simulink model "VCU_SW_1"  (R2023b)
settings: Solver=FixedStepDiscrete  StartTime=0.0  StopTime=inf  FixedStep=1e-2  RelTol=1e-3
PreLoadFcn:
  | RTWConfigurationCB('preloadfcn', bdroot);
InitFcn:
  | loadvar_ttc500
undefined symbols (not defined in the file): BrkPedalTypes, CabMovModeTypes, cFuseTempSensAcc_X, cFuseTempSensAcc_Y, cFuseTempSensVal_X, cFuseTempSensVal_Y, cTMSTempSensVal_X, cTMSTempSensVal_Y, cTransferCaseSpeedRatio, diag_state, DoorsPositionTypes, dP_filter_Y, DriverOccClassSystemTypes, ErrorValueTypes, fatal_error_callback, IO_ADC_NO_RANGE, LadderStatusTypes, pAnalogCabRotSensAcc, pAnalogCabRotSensMaxVolt, pAnalogCabRotSensMinVolt, pAnalogCabRotSensRange, pAnalogCabRotSensZeroVolt, pBrkActivePress, pCabTiltSensAcc, pCabTiltSensMaxCur, pCabTiltSensMinCur, pDistanceCorrection, pECANManual_BPNEnable, pECANManual_BPNEnabler_Flag, pFilterSensAccRes, pHDirMaxDiffFrq, pHDirSensHighLvl, pHDirSensLowLvl, pMainGearRatio, pMaxFilterSensRes, pMaxFirstPedalSensValue, pMaxFuseTempSensRes, pMaxPressLoss, pMaxPressSensCurrent, pMaxPressValue, pMaxPressValueHydMotAndPump, pMaxPressValueParkDrain, pMaxSecondPedalSensValue, pMaxTempSensVoltage, pMaxTempValue, pMaxTMSTempSensRes, pMinFilterSensRes, pMinFirstPedalSensValue, pMinFuseTempSensRes, pMinPressLoss, pMinPressSensCurrent, pMinPressValue, pMinSecondPedalSensValue, pMinTempSensVoltage, pMinTempValue, pMinTMSTempSensRes, pMotorRingTeethNum, pPedalSensAccuracyPct, pPedalSensAccuracyVolt, pPressLossTreshhold ... (+20)
libraries: TTlibrary x270, canmsglib x127, simulink x88
(part 10 of 19)

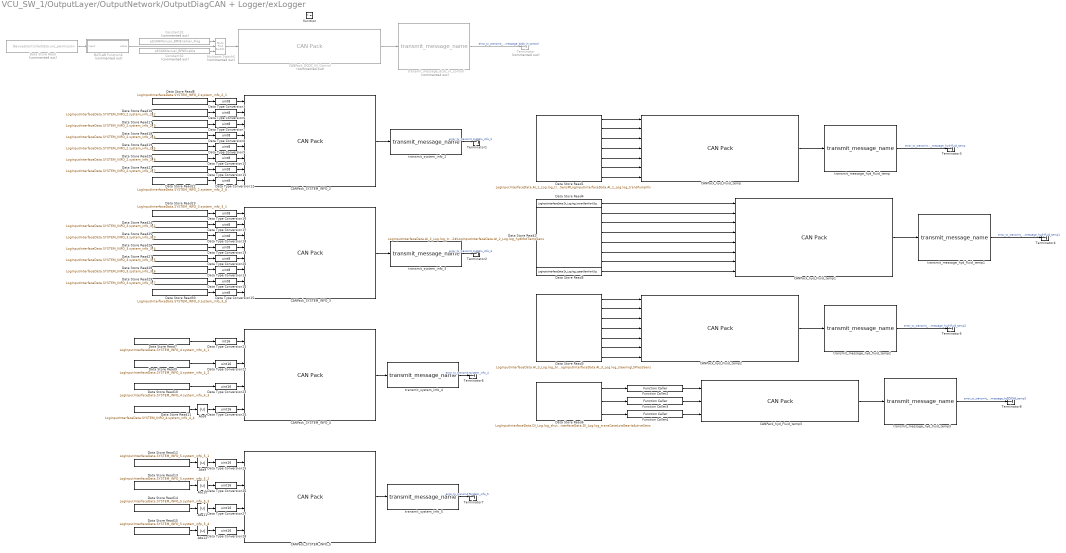
== system VCU_SW_1/OutputLayer/OutputNetwork/OutputDiagCAN + Logger/exLogger ==
  function : TriggerPort  TriggerType=function-call  VariantControl=Variant
  Abs{8..12} (5 alike) : Abs  SaturateOnIntegerOverflow=off
  CANPack_DCDC_IN_Control : canmsglib/CAN Pack  Commented=on  CANdbFile=C:\Users\shevchenko\Desktop\HerculesLittle\HerculesLittle\database\ElectricCAN.dbc  MsgList=(none)  MsgName=DCDC_IN_Control  MsgIDType=Extended (29-bit identifier)  MsgIdentifier=73  MsgLength=8  Remote=off  ApplyMinMax=off  BusOutput=on  SignalInfo={'BPN_Enable','0','1','LE','unsigned','Standard','0','1','0','0','1'}
      settings: DataFormat=CANdb specified signals
  CANPack_SYSTEM_INFO_2 : canmsglib/CAN Pack  MsgList=(none)  MsgName=SYSTEM_INFO_2  MsgIDType=Extended (29-bit identifier)  MsgIdentifier=419387898  MsgLength=8  Remote=off  ApplyMinMax=off  BusOutput=on  SignalInfo={ 'system_info_2_1', '0', '8', 'LE', 'unsigned', 'Standard', '0', '1', '0', '0', '255'; 'system_info_2_2', '8', '8', 'LE', 'unsigned', 'Standard', '0', '1', '0', '0', '255'; 'system_info_2_3', '16', '8', 'LE', 'unsigned', 'Standard', '0', '1', '0', '0', '255'; 'system_info_2_4', '24', '8', 'LE', 'unsigned', 'Standard', '0', '1', '0', '0', '255'; 'system_info_2_5', '32', '8', 'LE', 'unsigned', 'Standard', '0', '1', '0', '0', '255'; 'system_info_2_6', '40', '8', 'LE', 'unsigned', 'Standard', '0', '1', '0', '0', '255'; 'system_info_2_7', '48', '8', 'LE', 'unsigned', 'Standard', '0', '1', '0', '0', '255'; 'system_info_2_8', '56', '8', 'LE', 'unsigned', 'Standard', '0', '1', '0', '0', '255' }
      settings: DataFormat=manually specified signals
  CANPack_SYSTEM_INFO_3 : canmsglib/CAN Pack  MsgList=(none)  MsgName=SYSTEM_INFO_3  MsgIDType=Extended (29-bit identifier)  MsgIdentifier=419389690  MsgLength=8  Remote=off  ApplyMinMax=off  BusOutput=on  SignalInfo={ 'system_info_3_1', '0', '8', 'LE', 'unsigned', 'Standard', '0', '1', '0', '0', '255'; 'system_info_3_2', '8', '8', 'LE', 'unsigned', 'Standard', '0', '1', '0', '0', '255'; 'system_info_3_3', '16', '8', 'LE', 'unsigned', 'Standard', '0', '1', '0', '0', '255'; 'system_info_3_4', '24', '8', 'LE', 'unsigned', 'Standard', '0', '1', '0', '0', '255'; 'system_info_3_5', '32', '8', 'LE', 'unsigned', 'Standard', '0', '1', '0', '0', '255'; 'system_info_3_6', '40', '8', 'LE', 'unsigned', 'Standard', '0', '1', '0', '0', '255'; 'system_info_3_7', '48', '8', 'LE', 'unsigned', 'Standard', '0', '1', '0', '0', '255'; 'system_info_3_8', '56', '8', 'LE', 'unsigned', 'Standard', '0', '1', '0', '0', '255' }
      settings: DataFormat=manually specified signals
  CANPack_SYSTEM_INFO_4 : canmsglib/CAN Pack  MsgList=(none)  MsgName=SYSTEM_INFO_4  MsgIDType=Extended (29-bit identifier)  MsgIdentifier=419389946  MsgLength=8  Remote=off  ApplyMinMax=off  BusOutput=on  SignalInfo={ 'system_info_4_1', '0', '16', 'LE', 'unsigned', 'Standard', '0', '1', '-32768', '0', '32767'; 'system_info_4_2', '16', '16', 'LE', 'unsigned', 'Standard', '0', '1', '0', '0', '65535'; 'system_info_4_3', '32', '16', 'LE', 'unsigned', 'Standard', '0', '1', '0', '0', '65535'; 'system_info_4_4', '48', '16', 'LE', 'unsigned', 'Standard', '0', '1', '0', '0', '65535' }
      settings: DataFormat=manually specified signals
  CANPack_SYSTEM_INFO_5 : canmsglib/CAN Pack  MsgList=(none)  MsgName=SYSTEM_INFO_5  MsgIDType=Extended (29-bit identifier)  MsgIdentifier=419390202  MsgLength=8  Remote=off  ApplyMinMax=off  BusOutput=on  SignalInfo={ 'system_info_5_1', '0', '16', 'LE', 'unsigned', 'Standard', '0', '1', '0', '0', '65535'; 'system_info_5_2', '16', '16', 'LE', 'unsigned', 'Standard', '0', '1', '0', '0', '65535'; 'system_info_5_3', '32', '16', 'LE', 'unsigned', 'Standard', '0', '1', '0', '0', '65535'; 'system_info_5_4', '48', '16', 'LE', 'unsigned', 'Standard', '0', '1', '0', '0', '65535' }
      settings: DataFormat=manually specified signals
  CANPack_hyd_Fluid_temp : canmsglib/CAN Pack  MsgList=(none)  MsgName=Log_AI_1  MsgIDType=Extended (29-bit identifier)  MsgIdentifier=402657831  MsgLength=8  Remote=off  ApplyMinMax=off  BusOutput=on  SignalInfo={ 'TrHydPumpDirectSens', '24', '8', 'LE', 'unsigned', 'Standard', '0', '1', '0', '0', '255'; 'TrHydPumpFilterClogSens', '8', '8', 'LE', 'unsigned', 'Standard', '0', '2', '0', '0', '510'; 'TrHydPumpSpeedSens1', '32', '8', 'LE', 'unsigned', 'Standard', '0', '50', '0', '0', '12750'; 'TrHydPumpSpeedSens2', '16', '8', 'LE', 'unsigned', 'Standard', '0', '50', '0', '0', '12750'; 'TrHydPumpTempSens', '40', '8', 'LE', 'unsigned', 'Standard', '0', '10', '0', '0', '2550'; 'TrHydPumpWasherTiltSens', '0', '8', 'LE', 'unsigned', 'Standard', '0', '20', '0', '0', '5100'; 'TransmissionMotorHydDistr', '48', '8', 'LE', 'unsigned', 'Standard', '0', '4', '0', '0', '1020' }
      settings: DataFormat=manually specified signals
  CANPack_hyd_Fluid_temp1 : canmsglib/CAN Pack  MsgList=(none)  MsgName=Log_AI_2  MsgIDType=Extended (29-bit identifier)  MsgIdentifier=402658087  MsgLength=8  Remote=off  ApplyMinMax=off  BusOutput=on  SignalInfo={ 'LowerGeneratorSignal', '56', '8', 'LE', 'unsigned', 'Standard', '0', '1', '0', '0', '255'; 'TrHydMotDirectSens', '16', '8', 'LE', 'unsigned', 'Standard', '0', '1', '0', '0', '255'; 'TrHydMotPressLineInForwardSens', '40', '8', 'LE', 'unsigned', 'Standard', '0', '100', '0', '0', '25500'; 'TrHydMotPressLineInReverseSens', '32', '8', 'LE', 'unsigned', 'Standard', '0', '100', '0', '0', '25500'; 'TrHydMotSpeedSens1', '0', '8', 'LE', 'unsigned', 'Standard', '0', '50', '0', '0', '12750'; 'TrHydMotSpeedSens2', '8', '8', 'LE', 'unsigned', 'Standard', '0', '50', '0', '0', '12750'; 'TrHydMotTempSens', '24', '8', 'LE', 'unsigned', 'Standard', '0', '10', '0', '0', '2550'; 'UpperGeneratorSignal', '48', '8', 'LE', 'unsigned', 'Standard', '0', '1', '0', '0', '255' }
      settings: DataFormat=manually specified signals
  CANPack_hyd_Fluid_temp2 : canmsglib/CAN Pack  MsgList=(none)  MsgName=Log_AI_3_Brake  MsgIDType=Extended (29-bit identifier)  MsgIdentifier=402658599  MsgLength=8  Remote=off  ApplyMinMax=off  BusOutput=on  SignalInfo={ 'BrkFrontCircPressSens', '16', '8', 'LE', 'unsigned', 'Standard', '0', '100', '0', '0', '25500'; 'BrkFrontSupplyCircPressSens', '40', '8', 'LE', 'unsigned', 'Standard', '0', '100', '0', '0', '25500'; 'BrkParkCircPressSens', '48', '8', 'LE', 'unsigned', 'Standard', '0', '100', '0', '0', '25500'; 'BrkParkSupplyCircPressSens', '24', '8', 'LE', 'unsigned', 'Standard', '0', '100', '0', '0', '25500'; 'BrkRearCircPressSens', '8', '8', 'LE', 'unsigned', 'Standard', '0', '100', '0', '0', '25500'; 'BrkRearSupplyCircPressSens', '32', '8', 'LE', 'unsigned', 'Standard', '0', '100', '0', '0', '25500'; 'StrAndBrkLSPressSens', '0', '8', 'LE', 'unsigned', 'Standard', '0', '100', '0', '0', '25500' }
      settings: DataFormat=manually specified signals
  CANPack_hyd_Fluid_temp3 : canmsglib/CAN Pack  MsgList=(none)  MsgName=Log_DI  MsgIDType=Extended (29-bit identifier)  MsgIdentifier=402658343  MsgLength=8  Remote=off  ApplyMinMax=off  BusOutput=on  SignalInfo={ 'ShutdownButtonSignal', '16', '2', 'LE', 'unsigned', 'Standard', '0', '1', '0', '0', '3'; 'TCHighGearIsActiveSens', '0', '2', 'LE', 'unsigned', 'Standard', '0', '1', '0', '0', '3'; 'TCLowGearIsActiveSens', '8', '2', 'LE', 'unsigned', 'Standard', '0', '1', '0', '0', '3' }
      settings: DataFormat=manually specified signals
  Constant31 : Constant  Commented=on  Value=pECANManual_BPNEnabler_Flag
  Constant32 : Constant  Commented=on  Value=pECANManual_BPNEnable
  Data Store Read : DataStoreRead  Commented=on  DataStoreName=DevicesControllerData  DataStoreElements=DevicesControllerData.ovc_permission  IndexOptions=Index vector (dialog)  Indices=1  OutputSizes=1
  Data Store Read1 : DataStoreRead  DataStoreName=LogInputInterfaceData  DataStoreElements=LogInputInterfaceData.AI_1_Log.log_transmPumpDirSens#LogInputInterfaceData.AI_1_Log.log_filterClogSens#LogInputInterfaceData.AI_1_Log.log_transPumpSpdSensSig1#LogInputInterfaceData.AI_1_Log.log_transPumpSpdSensSig2#LogInputInterfaceData.AI_1_Log.log_transPumpTempSens#LogInputInterfaceData.AI_1_Log.log_washerTiltPumpTransSens#LogInputInterfaceData.AI_1_Log.log_transPumpVlv  IndexOptions=Index vector (dialog)  Indices=1  OutputSizes=1
  Data Store Read10 : DataStoreRead  DataStoreName=LogInputInterfaceData  DataStoreElements=LogInputInterfaceData.SYSTEM_INFO_4.system_info_4_3  IndexOptions=Index vector (dialog)  Indices=1  OutputSizes=1
  Data Store Read11 : DataStoreRead  DataStoreName=LogInputInterfaceData  DataStoreElements=LogInputInterfaceData.SYSTEM_INFO_4.system_info_4_4  IndexOptions=Index vector (dialog)  Indices=1  OutputSizes=1
  Data Store Read12 : DataStoreRead  DataStoreName=LogInputInterfaceData  DataStoreElements=LogInputInterfaceData.SYSTEM_INFO_5.system_info_5_1  IndexOptions=Index vector (dialog)  Indices=1  OutputSizes=1
  Data Store Read13 : DataStoreRead  DataStoreName=LogInputInterfaceData  DataStoreElements=LogInputInterfaceData.SYSTEM_INFO_5.system_info_5_2  IndexOptions=Index vector (dialog)  Indices=1  OutputSizes=1
  Data Store Read14 : DataStoreRead  DataStoreName=LogInputInterfaceData  DataStoreElements=LogInputInterfaceData.SYSTEM_INFO_5.system_info_5_3  IndexOptions=Index vector (dialog)  Indices=1  OutputSizes=1
  Data Store Read15 : DataStoreRead  DataStoreName=LogInputInterfaceData  DataStoreElements=LogInputInterfaceData.SYSTEM_INFO_5.system_info_5_4  IndexOptions=Index vector (dialog)  Indices=1  OutputSizes=1
  Data Store Read16 : DataStoreRead  DataStoreName=LogInputInterfaceData  DataStoreElements=LogInputInterfaceData.SYSTEM_INFO_2.system_info_2_2  IndexOptions=Index vector (dialog)  Indices=1  OutputSizes=1
  Data Store Read17 : DataStoreRead  DataStoreName=LogInputInterfaceData  DataStoreElements=LogInputInterfaceData.SYSTEM_INFO_2.system_info_2_3  IndexOptions=Index vector (dialog)  Indices=1  OutputSizes=1
  Data Store Read18 : DataStoreRead  DataStoreName=LogInputInterfaceData  DataStoreElements=LogInputInterfaceData.SYSTEM_INFO_2.system_info_2_4  IndexOptions=Index vector (dialog)  Indices=1  OutputSizes=1
  Data Store Read19 : DataStoreRead  DataStoreName=LogInputInterfaceData  DataStoreElements=LogInputInterfaceData.SYSTEM_INFO_2.system_info_2_5  IndexOptions=Index vector (dialog)  Indices=1  OutputSizes=1
  Data Store Read2 : DataStoreRead  DataStoreName=LogInputInterfaceData  DataStoreElements=LogInputInterfaceData.AI_2_Log.log_transmMotDirSens#LogInputInterfaceData.AI_2_Log.log_hydMotPressLinePressSens#LogInputInterfaceData.AI_2_Log.log_reverseTransmMotPessLinePressSens#LogInputInterfaceData.AI_2_Log.log_transmHydMotSpdSensSig1#LogInputInterfaceData.AI_2_Log.log_transmHydMotSpdSensSig2#LogInputInterfaceData.AI_2_Log.log_hydMotTempSens  IndexOptions=Index vector (dialog)  Indices=1  OutputSizes=1
  Data Store Read20 : DataStoreRead  DataStoreName=LogInputInterfaceData  DataStoreElements=LogInputInterfaceData.SYSTEM_INFO_2.system_info_2_6  IndexOptions=Index vector (dialog)  Indices=1  OutputSizes=1
  Data Store Read21 : DataStoreRead  DataStoreName=LogInputInterfaceData  DataStoreElements=LogInputInterfaceData.SYSTEM_INFO_2.system_info_2_7  IndexOptions=Index vector (dialog)  Indices=1  OutputSizes=1
  Data Store Read22 : DataStoreRead  DataStoreName=LogInputInterfaceData  DataStoreElements=LogInputInterfaceData.SYSTEM_INFO_2.system_info_2_8  IndexOptions=Index vector (dialog)  Indices=1  OutputSizes=1
  Data Store Read23 : DataStoreRead  DataStoreName=LogInputInterfaceData  DataStoreElements=LogInputInterfaceData.SYSTEM_INFO_3.system_info_3_1  IndexOptions=Index vector (dialog)  Indices=1  OutputSizes=1
  Data Store Read24 : DataStoreRead  DataStoreName=LogInputInterfaceData  DataStoreElements=LogInputInterfaceData.SYSTEM_INFO_3.system_info_3_2  IndexOptions=Index vector (dialog)  Indices=1  OutputSizes=1
  Data Store Read25 : DataStoreRead  DataStoreName=LogInputInterfaceData  DataStoreElements=LogInputInterfaceData.SYSTEM_INFO_3.system_info_3_3  IndexOptions=Index vector (dialog)  Indices=1  OutputSizes=1
  Data Store Read26 : DataStoreRead  DataStoreName=LogInputInterfaceData  DataStoreElements=LogInputInterfaceData.SYSTEM_INFO_3.system_info_3_4  IndexOptions=Index vector (dialog)  Indices=1  OutputSizes=1
  Data Store Read27 : DataStoreRead  DataStoreName=LogInputInterfaceData  DataStoreElements=LogInputInterfaceData.SYSTEM_INFO_3.system_info_3_5  IndexOptions=Index vector (dialog)  Indices=1  OutputSizes=1
  Data Store Read28 : DataStoreRead  DataStoreName=LogInputInterfaceData  DataStoreElements=LogInputInterfaceData.SYSTEM_INFO_3.system_info_3_6  IndexOptions=Index vector (dialog)  Indices=1  OutputSizes=1
  Data Store Read29 : DataStoreRead  DataStoreName=LogInputInterfaceData  DataStoreElements=LogInputInterfaceData.SYSTEM_INFO_3.system_info_3_7  IndexOptions=Index vector (dialog)  Indices=1  OutputSizes=1
  Data Store Read3 : DataStoreRead  DataStoreName=LogInputInterfaceData  DataStoreElements=LogInputInterfaceData.AI_3_Log.log_brkFrontCircPressSens#LogInputInterfaceData.AI_3_Log.log_brkSupplyFrontPressSens#LogInputInterfaceData.AI_3_Log.drainParkPressSens#LogInputInterfaceData.AI_3_Log.log_brkSupplyParkPressSens#LogInputInterfaceData.AI_3_Log.log_brkRearCircPressSens#LogInputInterfaceData.AI_3_Log.log_brkSupplyRearPressSens#LogInputInterfaceData.AI_3_Log.log_steeringLSPressSens  IndexOptions=Index vector (dialog)  Indices=1  OutputSizes=1
  Data Store Read30 : DataStoreRead  DataStoreName=LogInputInterfaceData  DataStoreElements=LogInputInterfaceData.SYSTEM_INFO_3.system_info_3_8  IndexOptions=Index vector (dialog)  Indices=1  OutputSizes=1
  Data Store Read4 : DataStoreRead  DataStoreName=LogInputInterfaceData  DataStoreElements=LogInputInterfaceData.DI_Log.log_lowerGenWorkSig  IndexOptions=Index vector (dialog)  Indices=1  OutputSizes=1
  Data Store Read5 : DataStoreRead  DataStoreName=LogInputInterfaceData  DataStoreElements=LogInputInterfaceData.DI_Log.log_upperGenWorkSig  IndexOptions=Index vector (dialog)  Indices=1  OutputSizes=1
  Data Store Read6 : DataStoreRead  DataStoreName=LogInputInterfaceData  DataStoreElements=LogInputInterfaceData.DI_Log.log_shutdownButtonSig#LogInputInterfaceData.DI_Log.log_transCaseHighGearIsActiveSens#LogInputInterfaceData.DI_Log.log_transCaseLowGearIsActiveSens  IndexOptions=Index vector (dialog)  Indices=1  OutputSizes=1
  Data Store Read7 : DataStoreRead  DataStoreName=LogInputInterfaceData  DataStoreElements=LogInputInterfaceData.SYSTEM_INFO_4.system_info_4_1  IndexOptions=Index vector (dialog)  Indices=1  OutputSizes=1
  Data Store Read8 : DataStoreRead  DataStoreName=LogInputInterfaceData  DataStoreElements=LogInputInterfaceData.SYSTEM_INFO_2.system_info_2_1  IndexOptions=Index vector (dialog)  Indices=1  OutputSizes=1
  Data Store Read9 : DataStoreRead  DataStoreName=LogInputInterfaceData  DataStoreElements=LogInputInterfaceData.SYSTEM_INFO_4.system_info_4_2  IndexOptions=Index vector (dialog)  Indices=1  OutputSizes=1
  Data Type Conversion{3,6..20} (16 alike) : DataTypeConversion  OutDataTypeStr=uint8  SaturateOnIntegerOverflow=off  RndMeth=Floor
  Data Type Conversion21 : DataTypeConversion  OutDataTypeStr=int16  SaturateOnIntegerOverflow=off  RndMeth=Floor
  Data Type Conversion{22..28} (7 alike) : DataTypeConversion  OutDataTypeStr=uint16  SaturateOnIntegerOverflow=off  RndMeth=Floor
  Function Caller2 : FunctionCaller  FunctionPrototype=rawValue = convDIOSttTypeToNum(enumValue)  InputArgumentSpecifications=<Enter example>  OutputArgumentSpecifications=<Enter example>
  Function Caller3 : FunctionCaller  FunctionPrototype=rawValue = convDIOSttTypeToNum(enumValue)  InputArgumentSpecifications=<Enter example>  OutputArgumentSpecifications=<Enter example>
  Function Caller4 : FunctionCaller  FunctionPrototype=rawValue = convDIOSttTypeToNum(enumValue)  InputArgumentSpecifications=<Enter example>  OutputArgumentSpecifications=<Enter example>
  MATLAB Function6 : MATLAB Function  Commented=on  TreatAsAtomicUnit=on
  Multiport Switch5 : MultiPortSwitch  Commented=on  DataPortOrder=Zero-based contiguous  Inputs=2  zeroidx=on  SaturateOnIntegerOverflow=off  InputSameDT=off
  Terminator : Terminator  Commented=on
  Terminator{1..8} (8 alike) : Terminator
  transmit_message_dcdc_in_control : TTlibrary/CAN/transmit_message_name  Commented=on  channel=IO_CAN_CHANNEL_0  id_format=IO_CAN_STD_FRAME  retranslation=off  io_error=on  sample_time=-1
      settings: SourceProductName=TT control 500 series
  transmit_message_hyd_fluid_temp{,1..3} (4 alike) : TTlibrary/CAN/transmit_message_name  channel=IO_CAN_CHANNEL_6  id_format=IO_CAN_EXT_FRAME  retranslation=off  io_error=on  sample_time=-1
      settings: SourceProductName=TT control 500 series
  transmit_system_info_{2..5} (4 alike) : TTlibrary/CAN/transmit_message_name  channel=IO_CAN_CHANNEL_6  id_format=IO_CAN_EXT_FRAME  retranslation=off  io_error=on  sample_time=-1
      settings: SourceProductName=TT control 500 series
  wires:
  Data Type Conversion27/1 -> CANPack_SYSTEM_INFO_5/3
  CANPack_SYSTEM_INFO_5/1 -> transmit_system_info_5/1
  Constant32/1 -> Multiport Switch5/3
  CANPack_DCDC_IN_Control/1 -> transmit_message_dcdc_in_control/1
  Data Type Conversion16/1 -> CANPack_SYSTEM_INFO_3/1
  transmit_system_info_3/1 -> Terminator2/1  "error_tx_transmit_system_info_3"
  Abs10/1 -> Data Type Conversion26/1
  Data Type Conversion10/1 -> CANPack_SYSTEM_INFO_2/6
  Data Type Conversion20/1 -> CANPack_SYSTEM_INFO_3/5
  Data Store Read2/6 -> CANPack_hyd_Fluid_temp1/7
  Data Type Conversion25/1 -> CANPack_SYSTEM_INFO_5/1
  CANPack_hyd_Fluid_temp1/1 -> transmit_message_hyd_fluid_temp1/1
  transmit_system_info_2/1 -> Terminator1/1  "error_tx_transmit_system_info_2"
  CANPack_SYSTEM_INFO_3/1 -> transmit_system_info_3/1
  Data Type Conversion8/1 -> CANPack_SYSTEM_INFO_2/4
  Data Type Conversion21/1 -> CANPack_SYSTEM_INFO_4/1
  Data Type Conversion7/1 -> CANPack_SYSTEM_INFO_2/3
  transmit_message_dcdc_in_control/1 -> Terminator/1  "error_tx_transmit_message_dcdc_in_control"
  Data Type Conversion9/1 -> CANPack_SYSTEM_INFO_2/5
  Data Type Conversion19/1 -> CANPack_SYSTEM_INFO_3/4
  Data Store Read6/2 -> Function Caller3/1
  Data Type Conversion17/1 -> CANPack_SYSTEM_INFO_3/2
  CANPack_hyd_Fluid_temp3/1 -> transmit_message_hyd_fluid_temp3/1
  Data Store Read1/3 -> CANPack_hyd_Fluid_temp/3
  transmit_message_hyd_fluid_temp1/1 -> Terminator4/1  "error_tx_transmit_message_hyd_fluid_temp1"
  transmit_message_hyd_fluid_temp/1 -> Terminator3/1  "error_tx_transmit_message_hyd_fluid_temp"
  Function Caller2/1 -> CANPack_hyd_Fluid_temp3/1
  Constant31/1 -> Multiport Switch5/1
  Data Type Conversion28/1 -> CANPack_SYSTEM_INFO_5/4
  Data Type Conversion3/1 -> CANPack_SYSTEM_INFO_2/1
  CANPack_SYSTEM_INFO_4/1 -> transmit_system_info_4/1
  Data Type Conversion15/1 -> CANPack_SYSTEM_INFO_3/8
  Data Store Read1/6 -> CANPack_hyd_Fluid_temp/6
  CANPack_hyd_Fluid_temp/1 -> transmit_message_hyd_fluid_temp/1
  Data Store Read5/1 -> CANPack_hyd_Fluid_temp1/8
  Data Type Conversion18/1 -> CANPack_SYSTEM_INFO_3/3
  Data Store Read9/1 -> Data Type Conversion22/1
  Data Type Conversion11/1 -> CANPack_SYSTEM_INFO_2/7
  CANPack_hyd_Fluid_temp2/1 -> transmit_message_hyd_fluid_temp2/1
  Data Store Read2/1 -> CANPack_hyd_Fluid_temp1/2
  Data Type Conversion23/1 -> CANPack_SYSTEM_INFO_4/3
  Data Store Read3/4 -> CANPack_hyd_Fluid_temp2/4
  Data Store Read3/7 -> CANPack_hyd_Fluid_temp2/7
  Data Store Read1/5 -> CANPack_hyd_Fluid_temp/5
  Data Store Read2/4 -> CANPack_hyd_Fluid_temp1/5
  transmit_message_hyd_fluid_temp2/1 -> Terminator5/1  "error_tx_transmit_message_hyd_fluid_temp2"
  Function Caller3/1 -> CANPack_hyd_Fluid_temp3/2
  Function Caller4/1 -> CANPack_hyd_Fluid_temp3/3
  Abs12/1 -> Data Type Conversion28/1
  Data Type Conversion22/1 -> CANPack_SYSTEM_INFO_4/2
  Data Type Conversion12/1 -> CANPack_SYSTEM_INFO_2/8
  Data Store Read3/6 -> CANPack_hyd_Fluid_temp2/6
  Data Store Read1/4 -> CANPack_hyd_Fluid_temp/4
  Data Store Read7/1 -> Data Type Conversion21/1
  Abs11/1 -> Data Type Conversion27/1
  CANPack_SYSTEM_INFO_2/1 -> transmit_system_info_2/1
  Data Store Read27/1 -> Data Type Conversion20/1
  Data Type Conversion24/1 -> CANPack_SYSTEM_INFO_4/4
  Data Store Read19/1 -> Data Type Conversion9/1
  Data Store Read20/1 -> Data Type Conversion10/1
  Data Type Conversion14/1 -> CANPack_SYSTEM_INFO_3/7
  Data Store Read13/1 -> Abs10/1
  transmit_system_info_5/1 -> Terminator7/1  "error_tx_transmit_system_info_5"
  Data Type Conversion13/1 -> CANPack_SYSTEM_INFO_3/6
  Data Store Read3/1 -> CANPack_hyd_Fluid_temp2/1
  Data Store Read4/1 -> CANPack_hyd_Fluid_temp1/1
  Data Store Read8/1 -> Data Type Conversion3/1
  Data Store Read15/1 -> Abs12/1
  Data Store Read3/5 -> CANPack_hyd_Fluid_temp2/5
  Data Store Read14/1 -> Abs11/1
  Data Store Read1/1 -> CANPack_hyd_Fluid_temp/1
  Data Store Read3/3 -> CANPack_hyd_Fluid_temp2/3
  Data Store Read1/7 -> CANPack_hyd_Fluid_temp/7
  Abs8/1 -> Data Type Conversion24/1
  Data Store Read12/1 -> Abs9/1
  Data Store Read16/1 -> Data Type Conversion6/1
  Data Store Read23/1 -> Data Type Conversion16/1
  Abs9/1 -> Data Type Conversion25/1
  Data Store Read2/3 -> CANPack_hyd_Fluid_temp1/4
  Data Store Read26/1 -> Data Type Conversion19/1
  Multiport Switch5/1 -> CANPack_DCDC_IN_Control/1
  Data Store Read22/1 -> Data Type Conversion12/1
  Data Store Read25/1 -> Data Type Conversion18/1
  Data Store Read21/1 -> Data Type Conversion11/1
  Data Store Read2/2 -> CANPack_hyd_Fluid_temp1/3
  Data Store Read17/1 -> Data Type Conversion7/1
  Data Store Read6/1 -> Function Caller2/1
  Data Store Read28/1 -> Data Type Conversion13/1
  Data Store Read1/2 -> CANPack_hyd_Fluid_temp/2
  Data Store Read6/3 -> Function Caller4/1
  Data Store Read29/1 -> Data Type Conversion14/1
  Data Store Read10/1 -> Data Type Conversion23/1
  MATLAB Function6/1(value) -> Multiport Switch5/2
  Data Store Read11/1 -> Abs8/1
  Data Store Read18/1 -> Data Type Conversion8/1
  transmit_system_info_4/1 -> Terminator6/1  "error_tx_transmit_system_info_4"
  transmit_message_hyd_fluid_temp3/1 -> Terminator8/1  "error_tx_transmit_message_hyd_fluid_temp3"
  Data Store Read/1 -> MATLAB Function6/1(input)
  Data Store Read3/2 -> CANPack_hyd_Fluid_temp2/2
  Data Store Read24/1 -> Data Type Conversion17/1
  Data Store Read30/1 -> Data Type Conversion15/1
  Data Store Read2/5 -> CANPack_hyd_Fluid_temp1/6
  Data Type Conversion26/1 -> CANPack_SYSTEM_INFO_5/2
  Data Type Conversion6/1 -> CANPack_SYSTEM_INFO_2/2

== system VCU_SW_1/OutputLayer/OutputNetwork/OutputEngCAN/SetEngCAN50msec ==
  function : TriggerPort  TriggerType=function-call  VariantControl=Variant
  Bus Selector1 : BusSelector  OutputSignals=ID  OutputAsBus=on
  CANPack_VCU_ECU_TSC1 : canmsglib/CAN Pack  MsgList=(none)  MsgName=VCU_ECU_TSC1  MsgIDType=Extended (29-bit identifier)  MsgIdentifier=201326599  MsgLength=8  Remote=off  ApplyMinMax=off  BusOutput=on  SignalInfo={ 'VCU_ECU_TSC1_ContPurp', '35', '5', 'LE', 'unsigned', 'Standard', '0', '1', '0', '0', '31'; 'VCU_ECU_TSC1_EngOverContMod', '0', '2', 'LE', 'unsigned', 'Standard', '0', '1', '0', '0', '3'; 'VCU_ECU_TSC1_EngReqSpContCond', '2', '2', 'LE', 'unsigned', 'Standard', '0', '1', '0', '0', '3'; 'VCU_ECU_TSC1_EngReqSpSL', '8', '16', 'LE', 'unsigned', 'Standard', '0', '0.125', '0', '0', '8031.875'; 'VCU_ECU_TSC1_EngReqTrqHR', '40', '4', 'LE', 'unsigned', 'Standard', '0', '0.125', '0', '0', '0.875'; 'VCU_ECU_TSC1_EngReqTrqTL', '24', '8', 'LE', 'unsigned', 'Standard', '0', '1', '-125', '-125', '125'; 'VCU_ECU_TSC1_MesChksum', '60', '4', 'LE', 'unsigned', 'Standard', '0', '1', '0', '0', '15'; 'VCU_ECU_TSC1_MessCnt', '56', '4', 'LE', 'unsigned', 'Standard', '0', '1', '0', '0', '15'; 'VCU_ECU_TSC1_OverContModPr', '4', '2', 'LE', 'unsigned', 'Standard', '0', '1', '0', '0', '3'; 'VCU_ECU_TSC1_TransRate', '32', '3', 'LE', 'unsigned', 'Standard', '0', '1', '0', '0', '7' }
      settings: DataFormat=manually specified signals
  Constant1 : Constant  Value=uint8(0)
  Data Store Read1 : DataStoreRead  DataStoreName=OutputNetworkData  DataStoreElements=OutputNetworkData.EngCAN.ContPurp#OutputNetworkData.EngCAN.EngOverContMod#OutputNetworkData.EngCAN.EngReqSpContCond#OutputNetworkData.EngCAN.EngReqSpSL#OutputNetworkData.EngCAN.EngReqTrqHR#OutputNetworkData.EngCAN.EngReqTrqTL#OutputNetworkData.EngCAN.MesChksum#OutputNetworkData.EngCAN.MessCnt#OutputNetworkData.EngCAN.OverContModPr#OutputNetworkData.EngCAN.TransRate  IndexOptions=Index vector (dialog)  Indices=1  OutputSizes=1
  Function-Call Subsystem1 : Subsystem  TreatAsAtomicUnit=on
  Less Than1 : RelationalOperator  Operator=>  OutDataTypeStr=boolean  RndMeth=Simplest  InputSameDT=off
  transmit_vcu_ecu_tsc1 : TTlibrary/CAN/transmit_message_name  channel=IO_CAN_CHANNEL_2  id_format=IO_CAN_EXT_FRAME  retranslation=off  io_error=on  sample_time=-1
      settings: SourceProductName=TT control 500 series
  wires:
  Less Than1/1 -> Function-Call Subsystem1/Enable
  Data Store Read1/2 -> CANPack_VCU_ECU_TSC1/2
  Data Store Read1/5 -> CANPack_VCU_ECU_TSC1/5
  Data Store Read1/1 -> CANPack_VCU_ECU_TSC1/1
  Constant1/1 -> Less Than1/2
  Data Store Read1/9 -> CANPack_VCU_ECU_TSC1/9
  Data Store Read1/8 -> CANPack_VCU_ECU_TSC1/8
  transmit_vcu_ecu_tsc1/1 -> Function-Call Subsystem1/2(error_sts), Less Than1/1  "error_tx_transmit_vcu_ecu_tsc1"
  Data Store Read1/6 -> CANPack_VCU_ECU_TSC1/6
  CANPack_VCU_ECU_TSC1/1 -> Bus Selector1/1, transmit_vcu_ecu_tsc1/1
  Data Store Read1/7 -> CANPack_VCU_ECU_TSC1/7
  Data Store Read1/10 -> CANPack_VCU_ECU_TSC1/10
  Data Store Read1/4 -> CANPack_VCU_ECU_TSC1/4
  Bus Selector1/1 -> Function-Call Subsystem1/1(In1)
  Data Store Read1/3 -> CANPack_VCU_ECU_TSC1/3

== system VCU_SW_1/OutputLayer/OutputNetwork/OutputHydCAN/SetHydCAN100msec ==
  note: См. outputFcn
  function : TriggerPort  TriggerType=function-call  VariantControl=Variant
  CANPack_hyd_Fluid_temp : canmsglib/CAN Pack  Commented=on  MsgList=(none)  MsgName=VEH_FLUID_TEMP  MsgIDType=Extended (29-bit identifier)  MsgIdentifier=419326202  MsgLength=1  Remote=off  ApplyMinMax=off  BusOutput=on  SignalInfo={ 'FluidTemp', '0', '8', 'LE', 'signed', 'Standard', '0', '1', '40', '-40', '120' }
      settings: DataFormat=manually specified signals
  Cabine1stLeftHydCylValve : Subsystem
  Cabine2ndRightHydCylValve : Subsystem
  CabineTurningValve : Subsystem
  Data Store Read : DataStoreRead  Commented=on  DataStoreName=OutputNetworkData  DataStoreElements=OutputNetworkData.HydCAN.fluidTemp  IndexOptions=Index vector (dialog)  Indices=1  OutputSizes=1
  Terminator : Terminator  Commented=on
  transmit_message_hyd_fluid_temp : TTlibrary/CAN/transmit_message_name  Commented=on  channel=IO_CAN_CHANNEL_0  id_format=IO_CAN_EXT_FRAME  retranslation=off  io_error=on  sample_time=-1
      settings: SourceProductName=TT control 500 series
  wires:
  transmit_message_hyd_fluid_temp/1 -> Terminator/1  "error_tx_transmit_message_hyd_fluid_temp"
  CANPack_hyd_Fluid_temp/1 -> transmit_message_hyd_fluid_temp/1
  Data Store Read/1 -> CANPack_hyd_Fluid_temp/1

== system VCU_SW_1/OutputLayer/OutputNetwork/OutputStrCAN/SetStrCAN100msec ==
  note: См. outputFcn
  function : TriggerPort  TriggerType=function-call  VariantControl=Variant
  CANPack_Str_Fluid_temp : canmsglib/CAN Pack  Commented=on  MsgList=(none)  MsgName=VEH_FLUID_TEMP  MsgIDType=Extended (29-bit identifier)  MsgIdentifier=419326202  MsgLength=1  Remote=off  ApplyMinMax=off  BusOutput=on  SignalInfo={ 'FluidTemp', '0', '8', 'LE', 'signed', 'Standard', '0', '1', '40', '-40', '120' }
      settings: DataFormat=manually specified signals
  CANPack_VLVCMD_STR1 : canmsglib/CAN Pack  MsgList=(none)  MsgName=VLVCMD_STR1  MsgIDType=Extended (29-bit identifier)  MsgIdentifier=217985274  MsgLength=3  Remote=off  ApplyMinMax=off  BusOutput=on  SignalInfo={ 'FailSafeModeCmdStr1', '22', '2', 'LE', 'unsigned', 'Standard', '0', '1', '0', '0', '3'; 'PortFlowCmdStr1', '0', '8', 'LE', 'unsigned', 'Standard', '0', '0.4', '0', '0', '100'; 'ValveStateStr1', '16', '4', 'LE', 'unsigned', 'Standard', '0', '1', '0', '0', '15' }
      settings: DataFormat=manually specified signals
  Data Store Read : DataStoreRead  Commented=on  DataStoreName=OutputNetworkData  DataStoreElements=OutputNetworkData.StrCAN.fluidTemp  IndexOptions=Index vector (dialog)  Indices=1  OutputSizes=1
  Data Store Read1 : DataStoreRead  DataStoreName=OutputNetworkData  DataStoreElements=OutputNetworkData.StrCAN.failSafeModeCmdStr1#OutputNetworkData.StrCAN.portFlowCmdStr1#OutputNetworkData.StrCAN.valveStateStr1  IndexOptions=Index vector (dialog)  Indices=1  OutputSizes=1
  Terminator : Terminator  Commented=on
  Terminator1 : Terminator
  transmit_message_str_fluid_temp : TTlibrary/CAN/transmit_message_name  Commented=on  channel=IO_CAN_CHANNEL_3  id_format=IO_CAN_EXT_FRAME  retranslation=off  io_error=on  sample_time=-1
      settings: SourceProductName=TT control 500 series
  transmit_message_vlvcmd_str1 : TTlibrary/CAN/transmit_message_name  channel=IO_CAN_CHANNEL_3  id_format=IO_CAN_EXT_FRAME  retranslation=off  io_error=on  sample_time=-1
      settings: SourceProductName=TT control 500 series
  wires:
  CANPack_Str_Fluid_temp/1 -> transmit_message_str_fluid_temp/1
  transmit_message_str_fluid_temp/1 -> Terminator/1  "error_tx_transmit_message_str_fluid_temp"
  Data Store Read/1 -> CANPack_Str_Fluid_temp/1
  Data Store Read1/1 -> CANPack_VLVCMD_STR1/1
  transmit_message_vlvcmd_str1/1 -> Terminator1/1  "error_tx_transmit_message_vlvcmd_str1"
  CANPack_VLVCMD_STR1/1 -> transmit_message_vlvcmd_str1/1
  Data Store Read1/2 -> CANPack_VLVCMD_STR1/2
  Data Store Read1/3 -> CANPack_VLVCMD_STR1/3

== system VCU_SW_1/logSignal/getListData/pageHighvoltageAppData/getListDataII1 ==
  getListDataII1 : TriggerPort  TriggerType=function-call  IsSimulinkFunction=on  FunctionName=getListDataII1  FunctionVisibility=scoped  VariantControl=(inherit)
  Constant : Constant  Value=uint8(5)
  Data Store Read1 : DataStoreRead  DataStoreName=sBmsCounter  IndexOptions=Index vector (dialog)  Indices=1  OutputSizes=1
  Data Store Read2 : DataStoreRead  DataStoreName=sChargeStopSignal  IndexOptions=Index vector (dialog)  Indices=1  OutputSizes=1
  Data Store Read3 : DataStoreRead  DataStoreName=sStopAll  IndexOptions=Index vector (dialog)  Indices=1  OutputSizes=1
  Data Store Read4 : DataStoreRead  DataStoreName=sBmsLocalState  IndexOptions=Index vector (dialog)  Indices=1  OutputSizes=1
  Demux11 : Demux  Outputs=2
  Function Caller : FunctionCaller  FunctionPrototype=data = getListData.splitIntoTwoBytes(value)  InputArgumentSpecifications=<Enter example>  OutputArgumentSpecifications=<Enter example>
  Ground : Ground
  Mux : Mux  Inputs=7
  data : ArgOut  DisableCoverage=on  OutDataTypeStr=uint8  PortDimensions=[1,7]  ArgumentName=data
  len : ArgOut  Port=2  OutDataTypeStr=uint8  ArgumentName=len
  wires:
  Data Store Read2/1 -> Mux/4
  Data Store Read3/1 -> Mux/5
  Demux11/2 -> Mux/3
  Data Store Read4/1 -> Mux/1
  Demux11/1 -> Mux/2
  Mux/1 -> data/1
  Constant/1 -> len/1
  Function Caller/1 -> Demux11/1
  Data Store Read1/1 -> Function Caller/1
  Ground/1 -> Mux/6, Mux/7

== system VCU_SW_1/logSignal/getListData/pageHighvoltageAppData/getListDataII10 ==
  getListDataII10 : TriggerPort  TriggerType=function-call  IsSimulinkFunction=on  FunctionName=getListDataII10  FunctionVisibility=scoped  VariantControl=(inherit)
  Constant : Constant  Value=uint8(4)
  Data Store Read1 : DataStoreRead  DataStoreName=sB5_modes_1  IndexOptions=Index vector (dialog)  Indices=1  OutputSizes=1
  Data Store Read2 : DataStoreRead  DataStoreName=sB5_mode_1  IndexOptions=Index vector (dialog)  Indices=1  OutputSizes=1
  Data Store Read5 : DataStoreRead  DataStoreName=sB5_ChargeMode  IndexOptions=Index vector (dialog)  Indices=1  OutputSizes=1
  Data Store Read6 : DataStoreRead  DataStoreName=sB5_power  IndexOptions=Index vector (dialog)  Indices=1  OutputSizes=1
  Ground : Ground
  Mux : Mux  Inputs=7
  data : ArgOut  DisableCoverage=on  OutDataTypeStr=uint8  PortDimensions=[1,7]  ArgumentName=data
  len : ArgOut  Port=2  OutDataTypeStr=uint8  ArgumentName=len
  wires:
  Mux/1 -> data/1
  Constant/1 -> len/1
  Data Store Read5/1 -> Mux/4
  Data Store Read6/1 -> Mux/3
  Data Store Read2/1 -> Mux/1
  Data Store Read1/1 -> Mux/2
  Ground/1 -> Mux/7, Mux/6, Mux/5

== system VCU_SW_1/logSignal/getListData/pageHighvoltageAppData/getListDataII11 ==
  getListDataII11 : TriggerPort  TriggerType=function-call  IsSimulinkFunction=on  FunctionName=getListDataII11  FunctionVisibility=scoped  VariantControl=(inherit)
  Constant : Constant  Value=uint8(5)
  Data Store Read1 : DataStoreRead  DataStoreName=sPlugUnlockPerm  IndexOptions=Index vector (dialog)  Indices=1  OutputSizes=1
  Data Store Read2 : DataStoreRead  DataStoreName=sChargeLocalState  IndexOptions=Index vector (dialog)  Indices=1  OutputSizes=1
  Data Store Read3 : DataStoreRead  DataStoreName=sChargePerm  IndexOptions=Index vector (dialog)  Indices=1  OutputSizes=1
  Data Store Read4 : DataStoreRead  DataStoreName=sPlugLockPerm  IndexOptions=Index vector (dialog)  Indices=1  OutputSizes=1
  Data Store Read5 : DataStoreRead  DataStoreName=sPrechargeComplete  IndexOptions=Index vector (dialog)  Indices=1  OutputSizes=1
  Ground : Ground
  Mux : Mux  Inputs=7
  data : ArgOut  DisableCoverage=on  OutDataTypeStr=uint8  PortDimensions=[1,7]  ArgumentName=data
  len : ArgOut  Port=2  OutDataTypeStr=uint8  ArgumentName=len
  wires:
  Mux/1 -> data/1
  Constant/1 -> len/1
  Data Store Read4/1 -> Mux/1
  Data Store Read1/1 -> Mux/2
  Data Store Read3/1 -> Mux/3
  Data Store Read2/1 -> Mux/4
  Data Store Read5/1 -> Mux/5
  Ground/1 -> Mux/6, Mux/7

== system VCU_SW_1/logSignal/getListData/pageHighvoltageAppData/getListDataII12 ==
  note: -32767 to 32767
  getListDataII12 : TriggerPort  TriggerType=function-call  IsSimulinkFunction=on  FunctionName=getListDataII12  FunctionVisibility=scoped  VariantControl=(inherit)
  Constant : Constant  Value=uint8(6)
  Data Store Read1 : DataStoreRead  DataStoreName=sAimTrq  IndexOptions=Index vector (dialog)  Indices=1  OutputSizes=1
  Data Store Read2 : DataStoreRead  DataStoreName=sT15GroupStt  IndexOptions=Index vector (dialog)  Indices=1  OutputSizes=1
  Data Store Read4 : DataStoreRead  DataStoreName=sInvLocalState  IndexOptions=Index vector (dialog)  Indices=1  OutputSizes=1
  Data Store Read5 : DataStoreRead  DataStoreName=sCurStepInv  IndexOptions=Index vector (dialog)  Indices=1  OutputSizes=1
  Data Type Conversion : DataTypeConversion  OutDataTypeStr=int32  SaturateOnIntegerOverflow=off  RndMeth=Floor
  Data Type Conversion1 : DataTypeConversion  OutDataTypeStr=uint16  SaturateOnIntegerOverflow=off  RndMeth=Floor
  Data Type Conversion2 : DataTypeConversion  OutDataTypeStr=int32  SaturateOnIntegerOverflow=off  RndMeth=Floor
  Data Type Conversion3 : DataTypeConversion  OutDataTypeStr=uint16  SaturateOnIntegerOverflow=off  RndMeth=Floor
  Demux1 : Demux  Outputs=2
  Demux11 : Demux  Outputs=2
  Function Caller : FunctionCaller  FunctionPrototype=data = getListData.splitIntoTwoBytes(value)  InputArgumentSpecifications=<Enter example>  OutputArgumentSpecifications=<Enter example>
  Function Caller1 : FunctionCaller  FunctionPrototype=data = getListData.splitIntoTwoBytes(value)  InputArgumentSpecifications=<Enter example>  OutputArgumentSpecifications=<Enter example>
  Ground : Ground
  Mux : Mux  Inputs=7
  Sum2 : Sum  Inputs=++|
  Sum3 : Sum  Inputs=|++
  offset : Constant  Value=int32(32767)
  data : ArgOut  DisableCoverage=on  OutDataTypeStr=uint8  PortDimensions=[1,7]  ArgumentName=data
  len : ArgOut  Port=2  OutDataTypeStr=uint8  ArgumentName=len
  wires:
  Ground/1 -> Mux/7
  Constant/1 -> len/1
  Mux/1 -> data/1
  Demux11/2 -> Mux/3
  Data Store Read1/1 -> Data Type Conversion2/1
  Function Caller/1 -> Demux11/1
  Demux11/1 -> Mux/2
  Data Store Read4/1 -> Mux/1
  Function Caller1/1 -> Demux1/1
  Demux1/2 -> Mux/5
  Demux1/1 -> Mux/4
  Data Store Read2/1 -> Mux/6
  Data Store Read5/1 -> Data Type Conversion/1
  Sum2/1 -> Data Type Conversion1/1
  Data Type Conversion1/1 -> Function Caller1/1
  Data Type Conversion/1 -> Sum2/2
  offset/1 -> Sum2/1, Sum3/2
  Sum3/1 -> Data Type Conversion3/1
  Data Type Conversion2/1 -> Sum3/1
  Data Type Conversion3/1 -> Function Caller/1

== system VCU_SW_1/logSignal/getListData/pageHighvoltageAppData/getListDataII2 ==
  getListDataII2 : TriggerPort  TriggerType=function-call  IsSimulinkFunction=on  FunctionName=getListDataII2  FunctionVisibility=scoped  VariantControl=(inherit)
  Constant : Constant  Value=uint8(4)
  Data Store Read1 : DataStoreRead  DataStoreName=sPermissibleChargeCurrent  IndexOptions=Index vector (dialog)  Indices=1  OutputSizes=1
  Data Store Read2 : DataStoreRead  DataStoreName=sPermissibleChargeVoltage  IndexOptions=Index vector (dialog)  Indices=1  OutputSizes=1
  Demux1 : Demux  Outputs=2
  Demux11 : Demux  Outputs=2
  Function Caller : FunctionCaller  FunctionPrototype=data = getListData.splitIntoTwoBytes(value)  InputArgumentSpecifications=<Enter example>  OutputArgumentSpecifications=<Enter example>
  Function Caller1 : FunctionCaller  FunctionPrototype=data = getListData.splitIntoTwoBytes(value)  InputArgumentSpecifications=<Enter example>  OutputArgumentSpecifications=<Enter example>
  Ground : Ground
  Mux : Mux  Inputs=7
  data : ArgOut  DisableCoverage=on  OutDataTypeStr=uint8  PortDimensions=[1,7]  ArgumentName=data
  len : ArgOut  Port=2  OutDataTypeStr=uint8  ArgumentName=len
  wires:
  Mux/1 -> data/1
  Constant/1 -> len/1
  Function Caller/1 -> Demux11/1
  Demux11/1 -> Mux/1
  Data Store Read1/1 -> Function Caller/1
  Demux11/2 -> Mux/2
  Demux1/1 -> Mux/3
  Function Caller1/1 -> Demux1/1
  Data Store Read2/1 -> Function Caller1/1
  Demux1/2 -> Mux/4
  Ground/1 -> Mux/5, Mux/6, Mux/7

== system VCU_SW_1/logSignal/getListData/pageHighvoltageAppData/getListDataII3 ==
  getListDataII3 : TriggerPort  TriggerType=function-call  IsSimulinkFunction=on  FunctionName=getListDataII3  FunctionVisibility=scoped  VariantControl=(inherit)
  Constant : Constant  Value=uint8(7)
  Data Store Read1 : DataStoreRead  DataStoreName=sCompressorPwm  IndexOptions=Index vector (dialog)  Indices=1  OutputSizes=1
  Data Store Read2 : DataStoreRead  DataStoreName=sTmsCounter  IndexOptions=Index vector (dialog)  Indices=1  OutputSizes=1
  Data Store Read3 : DataStoreRead  DataStoreName=sPumpPwm  IndexOptions=Index vector (dialog)  Indices=1  OutputSizes=1
  Data Store Read4 : DataStoreRead  DataStoreName=sFanControl  IndexOptions=Index vector (dialog)  Indices=1  OutputSizes=1
  Data Store Read5 : DataStoreRead  DataStoreName=sTmsLocalState  IndexOptions=Index vector (dialog)  Indices=1  OutputSizes=1
  Data Store Read6 : DataStoreRead  DataStoreName=sTmsCircleSelected  IndexOptions=Index vector (dialog)  Indices=1  OutputSizes=1
  Demux1 : Demux  Outputs=2
  Function Caller1 : FunctionCaller  FunctionPrototype=data = getListData.splitIntoTwoBytes(value)  InputArgumentSpecifications=<Enter example>  OutputArgumentSpecifications=<Enter example>
  Mux : Mux  Inputs=7
  data : ArgOut  DisableCoverage=on  OutDataTypeStr=uint8  PortDimensions=[1,7]  ArgumentName=data
  len : ArgOut  Port=2  OutDataTypeStr=uint8  ArgumentName=len
  wires:
  Mux/1 -> data/1
  Constant/1 -> len/1
  Function Caller1/1 -> Demux1/1
  Data Store Read2/1 -> Function Caller1/1
  Demux1/1 -> Mux/6
  Demux1/2 -> Mux/7
  Data Store Read1/1 -> Mux/1
  Data Store Read3/1 -> Mux/2
  Data Store Read4/1 -> Mux/3
  Data Store Read5/1 -> Mux/4
  Data Store Read6/1 -> Mux/5

== system VCU_SW_1/logSignal/getListData/pageHighvoltageAppData/getListDataII4 ==
  getListDataII4 : TriggerPort  TriggerType=function-call  IsSimulinkFunction=on  FunctionName=getListDataII4  FunctionVisibility=scoped  VariantControl=(inherit)
  Constant : Constant  Value=uint8(7)
  Data Store Read1 : DataStoreRead  DataStoreName=sCompressorCounter  IndexOptions=Index vector (dialog)  Indices=1  OutputSizes=1
  Data Store Read2 : DataStoreRead  DataStoreName=sValveControl  IndexOptions=Index vector (dialog)  Indices=1  OutputSizes=1
  Data Store Read3 : DataStoreRead  DataStoreName=sPreviousState  IndexOptions=Index vector (dialog)  Indices=1  OutputSizes=1
  Data Store Read4 : DataStoreRead  DataStoreName=sHeaterEnable  IndexOptions=Index vector (dialog)  Indices=1  OutputSizes=1
  Data Store Read5 : DataStoreRead  DataStoreName=sHeaterPowerControl  IndexOptions=Index vector (dialog)  Indices=1  OutputSizes=1
  Data Store Read6 : DataStoreRead  DataStoreName=sCompressorStart  IndexOptions=Index vector (dialog)  Indices=1  OutputSizes=1
  Demux11 : Demux  Outputs=2
  Function Caller : FunctionCaller  FunctionPrototype=data = getListData.splitIntoTwoBytes(value)  InputArgumentSpecifications=<Enter example>  OutputArgumentSpecifications=<Enter example>
  Mux : Mux  Inputs=7
  data : ArgOut  DisableCoverage=on  OutDataTypeStr=uint8  PortDimensions=[1,7]  ArgumentName=data
  len : ArgOut  Port=2  OutDataTypeStr=uint8  ArgumentName=len
  wires:
  Mux/1 -> data/1
  Constant/1 -> len/1
  Function Caller/1 -> Demux11/1
  Demux11/1 -> Mux/1
  Data Store Read1/1 -> Function Caller/1
  Demux11/2 -> Mux/2
  Data Store Read3/1 -> Mux/6
  Data Store Read2/1 -> Mux/7
  Data Store Read4/1 -> Mux/5
  Data Store Read5/1 -> Mux/4
  Data Store Read6/1 -> Mux/3

== system VCU_SW_1/logSignal/getListData/pageHighvoltageAppData/getListDataII5 ==
  getListDataII5 : TriggerPort  TriggerType=function-call  IsSimulinkFunction=on  FunctionName=getListDataII5  FunctionVisibility=scoped  VariantControl=(inherit)
  Constant : Constant  Value=uint8(7)
  Data Store Read1 : DataStoreRead  DataStoreName=sSelfCircCounter  IndexOptions=Index vector (dialog)  Indices=1  OutputSizes=1
  Data Store Read2 : DataStoreRead  DataStoreName=sCompressoSecondCircleEx  IndexOptions=Index vector (dialog)  Indices=1  OutputSizes=1
  Data Store Read3 : DataStoreRead  DataStoreName=sCompressorStartEx  IndexOptions=Index vector (dialog)  Indices=1  OutputSizes=1
  Data Store Read4 : DataStoreRead  DataStoreName=sCompressorOffEx  IndexOptions=Index vector (dialog)  Indices=1  OutputSizes=1
  Data Store Read5 : DataStoreRead  DataStoreName=sPumpSecondCircleEx  IndexOptions=Index vector (dialog)  Indices=1  OutputSizes=1
  Data Store Read6 : DataStoreRead  DataStoreName=sPumpOffEx  IndexOptions=Index vector (dialog)  Indices=1  OutputSizes=1
  Demux11 : Demux  Outputs=2
  Function Caller : FunctionCaller  FunctionPrototype=data = getListData.splitIntoTwoBytes(value)  InputArgumentSpecifications=<Enter example>  OutputArgumentSpecifications=<Enter example>
  Mux : Mux  Inputs=7
  data : ArgOut  DisableCoverage=on  OutDataTypeStr=uint8  PortDimensions=[1,7]  ArgumentName=data
  len : ArgOut  Port=2  OutDataTypeStr=uint8  ArgumentName=len
  wires:
  Mux/1 -> data/1
  Constant/1 -> len/1
  Function Caller/1 -> Demux11/1
  Demux11/1 -> Mux/1
  Data Store Read1/1 -> Function Caller/1
  Demux11/2 -> Mux/2
  Data Store Read2/1 -> Mux/7
  Data Store Read3/1 -> Mux/6
  Data Store Read4/1 -> Mux/5
  Data Store Read5/1 -> Mux/4
  Data Store Read6/1 -> Mux/3

== system VCU_SW_1/logSignal/getListData/pageHighvoltageAppData/getListDataII6 ==
  getListDataII6 : TriggerPort  TriggerType=function-call  IsSimulinkFunction=on  FunctionName=getListDataII6  FunctionVisibility=scoped  VariantControl=(inherit)
  Constant : Constant  Value=uint8(7)
  Data Store Read1 : DataStoreRead  DataStoreName=sEproCurrent  IndexOptions=Index vector (dialog)  Indices=1  OutputSizes=1
  Data Store Read2 : DataStoreRead  DataStoreName=sHeaterSecondCircleEx  IndexOptions=Index vector (dialog)  Indices=1  OutputSizes=1
  Data Store Read3 : DataStoreRead  DataStoreName=sHeaterTempEx  IndexOptions=Index vector (dialog)  Indices=1  OutputSizes=1
  Data Store Read4 : DataStoreRead  DataStoreName=sHeaterOffEx  IndexOptions=Index vector (dialog)  Indices=1  OutputSizes=1
  Data Store Read5 : DataStoreRead  DataStoreName=sEproStartCommand  IndexOptions=Index vector (dialog)  Indices=1  OutputSizes=1
  Data Store Read6 : DataStoreRead  DataStoreName=sEproPower  IndexOptions=Index vector (dialog)  Indices=1  OutputSizes=1
  Demux11 : Demux  Outputs=2
  Function Caller : FunctionCaller  FunctionPrototype=data = getListData.splitIntoTwoBytes(value)  InputArgumentSpecifications=<Enter example>  OutputArgumentSpecifications=<Enter example>
  Mux : Mux  Inputs=7
  data : ArgOut  DisableCoverage=on  OutDataTypeStr=uint8  PortDimensions=[1,7]  ArgumentName=data
  len : ArgOut  Port=2  OutDataTypeStr=uint8  ArgumentName=len
  wires:
  Mux/1 -> data/1
  Constant/1 -> len/1
  Data Store Read3/1 -> Mux/2
  Data Store Read4/1 -> Mux/1
  Data Store Read2/1 -> Mux/3
  Demux11/2 -> Mux/6
  Data Store Read1/1 -> Function Caller/1
  Function Caller/1 -> Demux11/1
  Demux11/1 -> Mux/5
  Data Store Read5/1 -> Mux/7
  Data Store Read6/1 -> Mux/4

== system VCU_SW_1/logSignal/getListData/pageHighvoltageAppData/getListDataII7 ==
  getListDataII7 : TriggerPort  TriggerType=function-call  IsSimulinkFunction=on  FunctionName=getListDataII7  FunctionVisibility=scoped  VariantControl=(inherit)
  Constant : Constant  Value=uint8(6)
  Data Store Read1 : DataStoreRead  DataStoreName=sPosIsolationResistence  IndexOptions=Index vector (dialog)  Indices=1  OutputSizes=1
  Data Store Read2 : DataStoreRead  DataStoreName=sNegIsolationResistence  IndexOptions=Index vector (dialog)  Indices=1  OutputSizes=1
  Data Store Read3 : DataStoreRead  DataStoreName=sMaxCellVoltage  IndexOptions=Index vector (dialog)  Indices=1  OutputSizes=1
  Demux1 : Demux  Outputs=2
  Demux11 : Demux  Outputs=2
  Demux2 : Demux  Outputs=2
  Function Caller : FunctionCaller  FunctionPrototype=data = getListData.splitIntoTwoBytes(value)  InputArgumentSpecifications=<Enter example>  OutputArgumentSpecifications=<Enter example>
  Function Caller1 : FunctionCaller  FunctionPrototype=data = getListData.splitIntoTwoBytes(value)  InputArgumentSpecifications=<Enter example>  OutputArgumentSpecifications=<Enter example>
  Function Caller2 : FunctionCaller  FunctionPrototype=data = getListData.splitIntoTwoBytes(value)  InputArgumentSpecifications=<Enter example>  OutputArgumentSpecifications=<Enter example>
  Ground : Ground
  Mux : Mux  Inputs=7
  data : ArgOut  DisableCoverage=on  OutDataTypeStr=uint8  PortDimensions=[1,7]  ArgumentName=data
  len : ArgOut  Port=2  OutDataTypeStr=uint8  ArgumentName=len
  wires:
  Demux11/2 -> Mux/2
  Data Store Read1/1 -> Function Caller/1
  Demux11/1 -> Mux/1
  Function Caller/1 -> Demux11/1
  Constant/1 -> len/1
  Mux/1 -> data/1
  Function Caller1/1 -> Demux1/1
  Demux1/1 -> Mux/3
  Data Store Read2/1 -> Function Caller1/1
  Demux1/2 -> Mux/4
  Demux2/2 -> Mux/6
  Data Store Read3/1 -> Function Caller2/1
  Demux2/1 -> Mux/5
  Function Caller2/1 -> Demux2/1
  Ground/1 -> Mux/7
